simulink model "Pendulo"  (R2024b)
settings: Solver=VariableStepAuto  StartTime=0.0  StopTime=100  MaxStep=0.01  RelTol=1e-3
InitFcn:
  | Ip = 0.079;
  | Mc = 0.7031;
  | lp = 0.3302;
  | Mp = 0.23;
  | Fc = 0;
  | Beq = 4.3;
  | g = 9.81;
  | Bp = 0.0024;

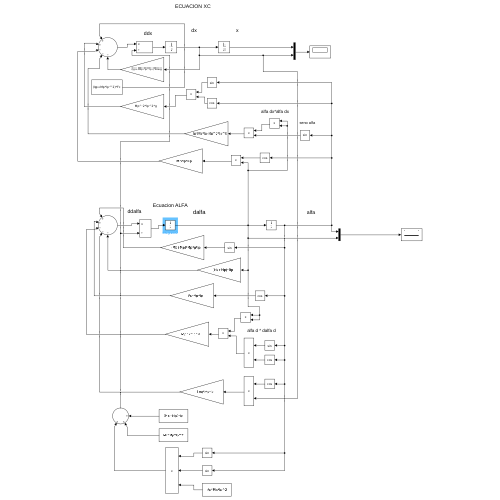
[thumbnail: Simulink's stored preview of the top-level diagram]
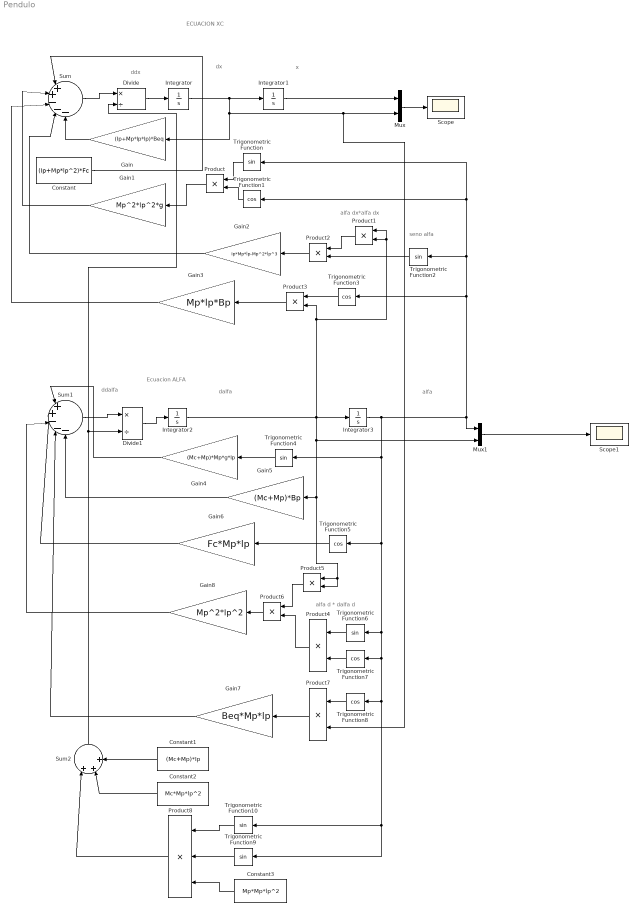
== system Pendulo ==
  note: alfa d * dalfa d
  note: seno alfa
  note: alfa dx*alfa dx
  note: alfa
  note: dalfa
  note: ddalfa
  note: Ecuacion ALFA
  note: x
  note: dx
  note: ddx
  note: ECUACION XC
  Constant : Constant  Value=(Ip+Mp*lp^2)*Fc
  Constant1 : Constant  Value=(Mc+Mp)*Ip
  Constant2 : Constant  Value=Mc*Mp*lp^2
  Constant3 : Constant  Value=Mp*Mp*lp^2
  Divide : Product  Inputs=*/
  Divide1 : Product  Inputs=*/
  Gain : Gain  Gain=(Ip+Mp*lp*lp)*Beq
  Gain1 : Gain  Gain=Mp^2*lp^2*g
  Gain2 : Gain  Gain=Ip*Mp*lp-Mp^2*lp^3
  Gain3 : Gain  Gain=Mp*lp*Bp
  Gain4 : Gain  Gain=(Mc+Mp)*Mp*g*lp
  Gain5 : Gain  Gain=(Mc+Mp)*Bp
  Gain6 : Gain  Gain=Fc*Mp*lp
  Gain7 : Gain  Gain=Beq*Mp*lp
  Gain8 : Gain  Gain=Mp^2*lp^2
  Integrator : Integrator
  Integrator1 : Integrator
  Integrator2 : Integrator
  Integrator3 : Integrator  InitialCondition=1*pi/180
  Mux : Mux  Inputs=2
  Mux1 : Mux  Inputs=2
  Product{,1..7} (8 alike) : Product
  Product8 : Product  Inputs=3
  Scope : Scope
  Scope1 : Scope
  Sum : Sum  Inputs=|++---
  Sum1 : Sum  Inputs=|++---
  Sum2 : Sum  Inputs=|+++
  Trigonometric Function{,2,4,6,9..10} (6 alike) : Trigonometry
  Trigonometric Function{1,3,5,7..8} (5 alike) : Trigonometry  Operator=cos
  wires:
  Constant/1 -> Sum/1
  Integrator/1 -> Gain/1, Product7/2, Mux/2, Integrator1/1
  Integrator1/1 -> Mux/1
  Mux/1 -> Scope/1
  Gain/1 -> Sum/5
  Integrator2/1 -> Product5/2, Product5/1, Gain5/1, Mux1/2, Product1/1, Product1/2, Product3/2, Integrator3/1
  Mux1/1 -> Scope1/1
  Integrator3/1 -> Trigonometric Function9/1, Trigonometric Function10/1, Trigonometric Function8/1, Trigonometric Function7/1, Trigonometric Function6/1, Trigonometric Function5/1, Trigonometric Function4/1, Trigonometric Function3/1, Trigonometric Function1/1, Trigonometric Function/1, Trigonometric Function2/1, Mux1/1
  Trigonometric Function/1 -> Product/1
  Trigonometric Function1/1 -> Product/2
  Product/1 -> Gain1/1
  Gain1/1 -> Sum/2
  Product1/1 -> Product2/1
  Trigonometric Function2/1 -> Product2/2
  Product2/1 -> Gain2/1
  Gain2/1 -> Sum/4
  Trigonometric Function3/1 -> Product3/1
  Product3/1 -> Gain3/1
  Gain3/1 -> Sum/3
  Trigonometric Function4/1 -> Gain4/1
  Gain4/1 -> Sum1/1
  Gain5/1 -> Sum1/5
  Trigonometric Function5/1 -> Gain6/1
  Gain6/1 -> Sum1/2
  Trigonometric Function6/1 -> Product4/1
  Trigonometric Function7/1 -> Product4/2
  Product5/1 -> Product6/1
  Product4/1 -> Product6/2
  Product6/1 -> Gain8/1
  Gain8/1 -> Sum1/3
  Trigonometric Function8/1 -> Product7/1
  Product7/1 -> Gain7/1
  Gain7/1 -> Sum1/4
  Constant1/1 -> Sum2/3
  Constant2/1 -> Sum2/2
  Trigonometric Function10/1 -> Product8/1
  Trigonometric Function9/1 -> Product8/2
  Constant3/1 -> Product8/3
  Product8/1 -> Sum2/1
  Divide/1 -> Integrator/1
  Sum/1 -> Divide/1
  Sum2/1 -> Divide/2, Divide1/2
  Divide1/1 -> Integrator2/1
  Sum1/1 -> Divide1/1
